simulink model "mobile_model_paths"  (R2023b)
settings: Solver=FixedStepAuto  StartTime=0.0  StopTime=100  FixedStep=dt  RelTol=1e-3
values from neighbouring files (symbols this model uses):
  dt = T / N    (= 0.1)    [mobile_paths.m]
libraries: robotmobilelib x1
settings Model: Creator=adnan  LastModifiedBy=adnan

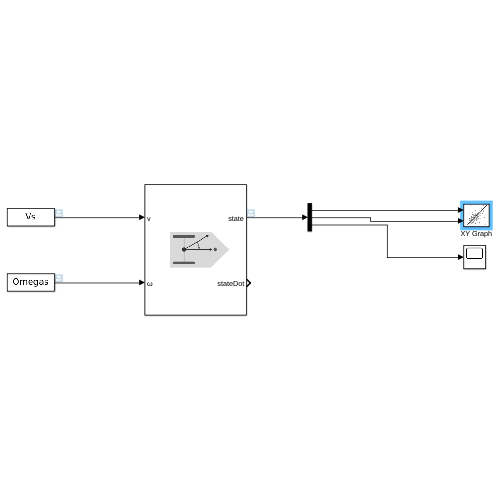
[thumbnail: Simulink's stored preview of the top-level diagram]
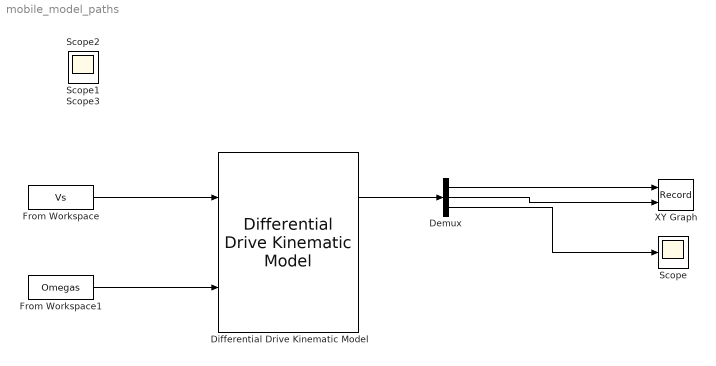
== system mobile_model_paths ==
  Demux : Demux  Outputs=3
  Differential Drive Kinematic Model : robotmobilelib/Differential Drive Kinematic Model  VehicleInputs=Vehicle Speed & Heading Angular Velocity  WheelRadius=1  WheelSpeedRange=[-inf inf]  TrackWidth=0.2  InitialState=[0; 0; 0]  SimulateUsing=Code generation
  From Workspace : FromWorkspace  VariableName=Vs  OutDataTypeStr=double  SampleTime=dt
  From Workspace1 : FromWorkspace  VariableName=Omegas  SampleTime=dt
  Scope{,1..3} (4 alike) : Scope
  XY Graph : Record  FileSettingsInternal="{\"entries\":[{\"content\":{\"excelSettings\":{\"content\":{},\"type\":\"Streamout.ExcelSettings\"}},\"type\":\"Streamout.FileSettingStorage\",\"uuid\":\"\"}],\"packageUris\":[\"http:\\/\\/schema.mathworks.com\\/mf0\\/streamout_blocks\\/R2020a\"],\"version\":\"1.0\"}"  Layout=[1 1]  SignalsInternal="{\"entries\":[{\"content\":{\"signals\":[{\"content\":{\"blockPath\":[],\"dimensions\":[1],\"domain\":\"\",\"lineColor\":\"#0072bd\",\"plots\":[1],\"port\":1,\"sid\":[\"\"],\"signalID\":777,\"signalName\":\"Demux:1\"},\"type\":\"RecordBlkView.Signal\",\"uuid\":\"\"},{\"content\":{\"blockPath\":[],\"dimensions\":[1],\"domain\":\"\",\"lineColor\":\"#0072bd\",\"plots\":[1],\"port\":2,\"sid\":[\"\"],\"signalID\":781,\"signalName\":\"Demux:2\"},\"type\":\"RecordBlkView.Signal\",\"uuid\":\"\"}]},\"type\":\"RecordBlkView.InputSignals\",\"uuid\":\"\"}],\"packageUris\":[\"http:\\/\\/schema.mathworks.com\\/mf0\\/streamout_blocks\\/R2020a\"],\"version\":\"1.0\"}"  VisualizationBindings="{\"xyplotplugin\":{\"info\":[{\"series\":[{\"bindingParametersList\":[{\"parameter\":\"X-Axis\",\"signalID\":777,\"signalName\":\"Demux:1\"},{\"parameter\":\"Y-Axis\",\"signalID\":781,\"signalName\":\"Demux:2\"}],\"seriesID\":53989}],\"subplotID\":1}]}}"  CompatibilityTag=XY
  wires:
  Differential Drive Kinematic Model/1 -> Demux/1
  Demux/1 -> XY Graph/1
  Demux/2 -> XY Graph/2
  Demux/3 -> Scope/1
  From Workspace/1 -> Differential Drive Kinematic Model/1
  From Workspace1/1 -> Differential Drive Kinematic Model/2
